simulink model "sampleModel1407_1_sub_sub"  (R2023a)
settings: Solver=VariableStepAuto  StartTime=0.0  StopTime=10.0  RelTol=1e-3
libraries: hdlsllib x1
settings Model: Creator=user1  LastModifiedBy=user1
settings OptimizationCC: BlockReduction=off  ConditionallyExecuteInputs=off

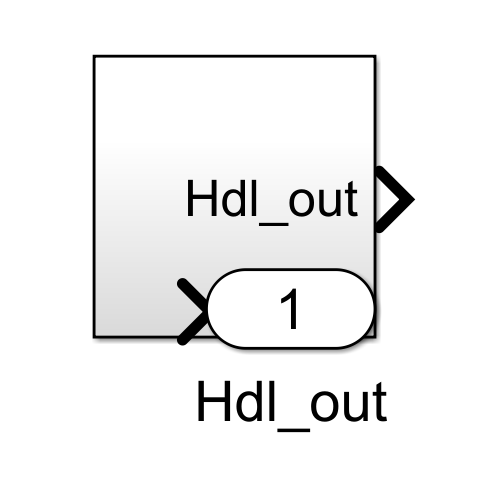
[thumbnail: Simulink's stored preview of the top-level diagram]
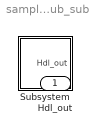
== system sampleModel1407_1_sub_sub ==
  Subsystem : Subsystem
  Hdl_out : Outport  OutDataTypeStr=uint8

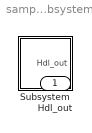
== system sampleModel1407_1_sub_sub/Subsystem ==
  Subsystem : Subsystem
  Hdl_out : Outport  OutDataTypeStr=uint8

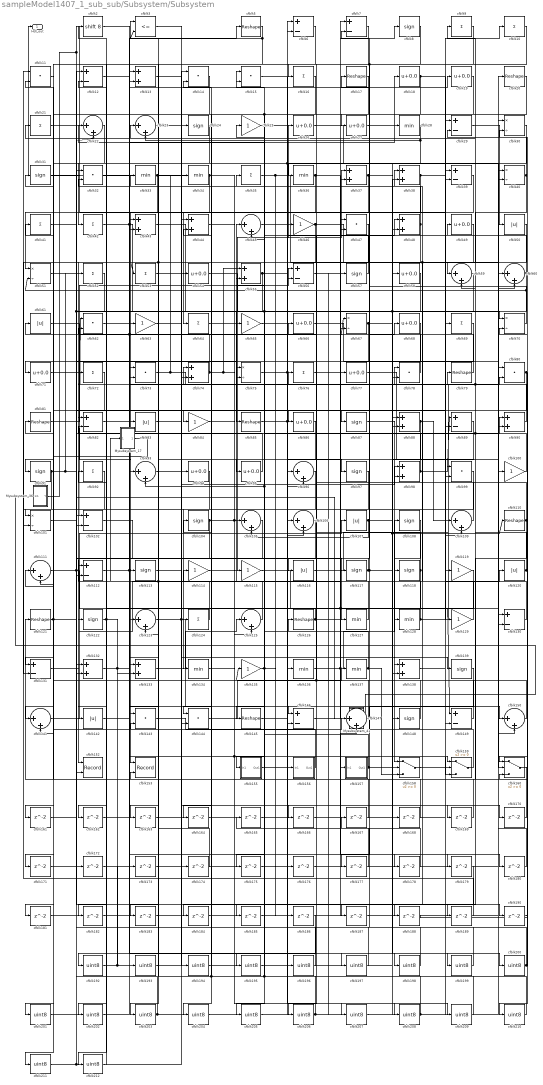
== system sampleModel1407_1_sub_sub/Subsystem/Subsystem ==
  Mysubsystem_17 : Subsystem  TreatAsAtomicUnit=on  RTWFcnName=Mysubsystem_17
      settings: RTWFcnNameOpts=User specified  RTWFileNameOpts=Use function name
  Mysubsystem_36 : Subsystem  TreatAsAtomicUnit=on  RTWFcnName=Mysubsystem_36
      settings: RTWFcnNameOpts=User specified  RTWFileNameOpts=Use function name
  Mysubsystem_41 : Subsystem  TreatAsAtomicUnit=on  RTWFcnName=Mysubsystem_41
      settings: RTWFcnNameOpts=User specified  RTWFileNameOpts=Use function name
  cfblk{9..10,16,21,35,41..42,52..53,64,69,72,76,92,124} (15 alike) : Sum  Inputs=+  OutDataTypeStr=uint8
  cfblk{25,46,63,65,84,100,114..115,119,129,135} (11 alike) : Gain  OutDataTypeStr=uint8
  cfblk{30,40,51,67,70,75,101} (7 alike) : Product  Inputs=*/  OutDataTypeStr=uint8  RndMeth=Zero  SaturateOnIntegerOverflow=on
  cfblk{6..7,12,29,39,56,82,89,102,112,130..131,146,149} (14 alike) : Sum  Inputs=+-  OutDataTypeStr=uint8
  cfblk{8,24,31,57,87,91,97,104,108,113,117..118,122,139,148} (15 alike) : Signum
  cfblk{22..23,45,59..60,93,96,105..106,109,111,123,125,141,147,150} (16 alike) : Sum  Inputs=|++  OutDataTypeStr=uint8
  cfblk{50,61,83,107,116,120,142} (7 alike) : Abs  OutDataTypeStr=uint8  SaturateOnIntegerOverflow=off
  cfblk{11,14..15,32,47,62,73,78,80,99,143..144} (12 alike) : DotProduct  OutDataTypeStr=uint8
  cfblk{5,17,20,79,81,85,110,121,126,145} (10 alike) : Reshape
  cfblk{28,33..34,36,127..128,134,136..137} (9 alike) : MinMax  OutDataTypeStr=uint8
  cfblk{13,37..38,43..44,48,55,74,88,90,98,132..133,138} (14 alike) : Sum  OutDataTypeStr=uint8
  cfblk152 : Record  FileSettingsInternal="{\"entries\":[{\"content\":{\"excelSettings\":{\"content\":{},\"type\":\"Streamout.ExcelSettings\"}},\"type\":\"Streamout.FileSettingStorage\",\"uuid\":\"\"}],\"packageUris\":[\"http:\\/\\/schema.mathworks.com\\/mf0\\/streamout_blocks\\/R2020a\"],\"version\":\"1.0\"}"  Layout=[1 1]  SignalsInternal="{\"entries\":[{\"content\":{\"signals\":[{\"content\":{\"blockPath\":[],\"dimensions\":[1],\"domain\":\"\",\"lineColor\":\"#a2142f\",\"plots\":[1],\"port\":1,\"signalID\":12907,\"signalName\":\"cfblk99\"},\"type\":\"RecordBlkView.Signal\",\"uuid\":\"\"},{\"content\":{\"blockPath\":[],\"dimensions\":[1],\"domain\":\"\",\"lineColor\":\"#139fff\",\"plots\":[1],\"port\":2,\"signalID\":12910,\"signalName\":\"cfblk20\"},\"type\":\"RecordBlkView.Signal\",\"uuid\":\"\"}]},\"type\":\"RecordBlkView.InputSignals\",\"uuid\":\"\"}],\"packageUris\":[\"http:\\/\\/schema.mathworks.com\\/mf0\\/streamout_blocks\\/R2020a\"],\"version\":\"1.0\"}"  VisualizationBindings="{\"xyplotplugin\":{\"info\":[{\"series\":[{\"bindingParametersList\":[{\"parameter\":\"X-Axis\",\"signalID\":12907,\"signalName\":\"cfblk99\"},{\"parameter\":\"Y-Axis\",\"signalID\":12910,\"signalName\":\"cfblk20\"}],\"seriesID\":1819}],\"subplotID\":1}]}}"  CompatibilityTag=XY  st=-1
  cfblk153 : Record  FileSettingsInternal="{\"entries\":[{\"content\":{\"excelSettings\":{\"content\":{},\"type\":\"Streamout.ExcelSettings\"}},\"type\":\"Streamout.FileSettingStorage\",\"uuid\":\"\"}],\"packageUris\":[\"http:\\/\\/schema.mathworks.com\\/mf0\\/streamout_blocks\\/R2020a\"],\"version\":\"1.0\"}"  Layout=[1 1]  SignalsInternal="{\"entries\":[{\"content\":{\"signals\":[{\"content\":{\"blockPath\":[],\"dimensions\":[1],\"domain\":\"\",\"lineColor\":\"#a2142f\",\"plots\":[1],\"port\":1,\"signalID\":12899,\"signalName\":\"cfblk47\"},\"type\":\"RecordBlkView.Signal\",\"uuid\":\"\"},{\"content\":{\"blockPath\":[],\"dimensions\":[1],\"domain\":\"\",\"lineColor\":\"#139fff\",\"plots\":[1],\"port\":2,\"signalID\":12902,\"signalName\":\"cfblk208\"},\"type\":\"RecordBlkView.Signal\",\"uuid\":\"\"}]},\"type\":\"RecordBlkView.InputSignals\",\"uuid\":\"\"}],\"packageUris\":[\"http:\\/\\/schema.mathworks.com\\/mf0\\/streamout_blocks\\/R2020a\"],\"version\":\"1.0\"}"  VisualizationBindings="{\"xyplotplugin\":{\"info\":[{\"series\":[{\"bindingParametersList\":[{\"parameter\":\"X-Axis\",\"signalID\":12899,\"signalName\":\"cfblk47\"},{\"parameter\":\"Y-Axis\",\"signalID\":12902,\"signalName\":\"cfblk208\"}],\"seriesID\":54978}],\"subplotID\":1}]}}"  CompatibilityTag=XY  st=-1
  cfblk155 : Subsystem
      settings: LibrarySourceBlock=|
      | hdlsllib/Ports &
      | Subsystems/Subsystem
  cfblk156 : Subsystem
      settings: LibrarySourceBlock=|
      | hdlsllib/Ports &
      | Subsystems/Subsystem
  cfblk157 : Subsystem
      settings: LibrarySourceBlock=|
      | hdlsllib/Ports &
      | Subsystems/Subsystem
  cfblk158 : Switch  OutDataTypeStr=uint8  SaturateOnIntegerOverflow=off  InputSameDT=off
  cfblk159 : Switch  OutDataTypeStr=uint8  SaturateOnIntegerOverflow=off  InputSameDT=off
  cfblk160 : Switch  OutDataTypeStr=uint8  SaturateOnIntegerOverflow=off  InputSameDT=off
  cfblk{161..190} (30 alike) : Delay  SampleTime=1
  cfblk{18..19,26..27,49,54,58,66,68,71,77,86,94..95} (14 alike) : Bias  Bias=0.0  SaturateOnIntegerOverflow=off
  cfblk{192..212} (21 alike) : DataTypeConversion  OutDataTypeStr=uint8  SaturateOnIntegerOverflow=off  RndMeth=Floor
  cfblk2 : ArithShift  BitShiftNumber=8
  cfblk3 : RelationalOperator  Operator=<=  OutDataTypeStr=boolean  InputSameDT=off
  Hdl_out : Outport  OutDataTypeStr=uint8
  wires:
  Mysubsystem_41/1(Out1) -> Mysubsystem_36/1(In1)
  Mysubsystem_36/1(Y) -> cfblk64/1, cfblk75/1
  Mysubsystem_17/1(Out1) -> cfblk161/1
  cfblk125/1 -> Mysubsystem_17/1(In1)
  cfblk212/1 -> cfblk92/1
  cfblk16/1 -> cfblk212/1
  cfblk211/1 -> cfblk22/2, cfblk94/1
  cfblk210/1 -> cfblk44/2
  cfblk209/1 -> cfblk44/1
  cfblk165/1 -> cfblk209/1
  cfblk208/1 -> cfblk14/2, cfblk153/2, cfblk75/2, cfblk20/1
  cfblk207/1 -> cfblk69/1
  cfblk206/1 -> cfblk123/2, cfblk57/1
  cfblk205/1 -> cfblk96/2
  cfblk204/1 -> cfblk96/1
  cfblk179/1 -> cfblk204/1
  cfblk203/1 -> cfblk132/1, cfblk148/1
  cfblk202/1 -> cfblk13/2
  cfblk186/1 -> cfblk202/1
  cfblk201/1 -> cfblk13/1
  cfblk11/1 -> cfblk201/1
  cfblk200/1 -> cfblk165/1, cfblk30/2
  cfblk199/1 -> cfblk65/1
  cfblk198/1 -> cfblk167/1
  cfblk65/1 -> cfblk198/1
  cfblk197/1 -> cfblk12/2
  cfblk196/1 -> cfblk12/1
  cfblk145/1 -> cfblk196/1
  cfblk195/1 -> cfblk168/1
  cfblk12/1 -> cfblk195/1
  cfblk194/1 -> cfblk106/2
  cfblk3/1 -> cfblk194/1
  cfblk193/1 -> cfblk106/1
  cfblk192/1 -> cfblk174/1, cfblk173/1
  cfblk190/1 -> cfblk160/3
  cfblk189/1 -> cfblk11/1
  cfblk188/1 -> cfblk160/1
  cfblk187/1 -> cfblk39/1
  cfblk185/1 -> cfblk88/1
  cfblk184/1 -> cfblk60/1
  cfblk183/1 -> cfblk144/2
  cfblk182/1 -> cfblk147/2
  cfblk119/1 -> cfblk182/1
  cfblk181/1 -> cfblk80/1
  cfblk180/1 -> cfblk40/1
  cfblk63/1 -> cfblk180/1
  cfblk178/1 -> cfblk15/2
  cfblk76/1 -> cfblk178/1
  cfblk177/1 -> cfblk45/2
  cfblk139/1 -> cfblk177/1
  cfblk176/1 -> cfblk109/2
  cfblk175/1 -> cfblk158/2
  cfblk174/1 -> cfblk143/2
  cfblk173/1 -> cfblk30/1
  cfblk172/1 -> cfblk62/2
  cfblk51/1 -> cfblk172/1
  cfblk171/1 -> cfblk74/2
  cfblk24/1 -> cfblk171/1
  cfblk170/1 -> cfblk59/2
  cfblk169/1 -> cfblk111/1
  cfblk168/1 -> cfblk14/1
  cfblk167/1 -> cfblk102/1
  cfblk166/1 -> cfblk149/2
  cfblk83/1 -> cfblk166/1
  cfblk164/1 -> cfblk56/2
  cfblk163/1 -> cfblk48/2
  cfblk105/1 -> cfblk163/1
  cfblk162/1 -> cfblk73/1
  cfblk161/1 -> cfblk32/1
  cfblk93/1 -> cfblk138/1
  cfblk121/1 -> cfblk81/1, cfblk90/2
  cfblk107/1 -> cfblk105/2, cfblk170/1
  cfblk66/1 -> cfblk150/2
  cfblk17/1 -> cfblk36/1
  cfblk39/1 -> cfblk142/1
  cfblk23/1 -> cfblk24/1
  cfblk86/1 -> cfblk133/1
  cfblk33/1 -> cfblk43/2, cfblk88/2
  cfblk137/1 -> cfblk25/1, cfblk93/2, cfblk158/3
  cfblk71/1 -> cfblk38/2
  cfblk27/1 -> cfblk18/1
  cfblk89/1 -> cfblk95/1
  cfblk48/1 -> cfblk32/2, cfblk124/1
  cfblk148/1 -> cfblk135/1, cfblk126/1
  cfblk25/1 -> cfblk97/1
  cfblk135/1 -> cfblk175/1, cfblk176/1
  cfblk40/1 -> cfblk59/1, cfblk29/2
  cfblk91/1 -> Mysubsystem_41/1(In1), cfblk52/1, cfblk131/2
  cfblk43/1 -> cfblk105/1
  cfblk64/1 -> cfblk26/1
  cfblk53/1 -> cfblk99/2
  cfblk19/1 -> cfblk54/1, cfblk205/1
  cfblk100/1 -> cfblk49/1, cfblk46/1
  cfblk144/1 -> cfblk137/1
  cfblk13/1 -> cfblk200/1
  cfblk156/1(Out1) -> cfblk41/1
  cfblk67/1 -> cfblk99/1, cfblk145/1
  cfblk106/1 -> cfblk192/1
  cfblk57/1 -> cfblk22/1
  cfblk5/1 -> cfblk73/2, cfblk3/2
  cfblk9/1 -> cfblk87/1, cfblk112/1
  cfblk58/1 -> cfblk117/1
  cfblk84/1 -> cfblk115/1
  cfblk80/1 -> cfblk162/1, cfblk210/1
  cfblk77/1 -> cfblk130/1
  cfblk114/1 -> cfblk29/1
  cfblk20/1 -> cfblk152/2
  cfblk129/1 -> cfblk104/1
  cfblk90/1 -> cfblk78/1
  cfblk113/1 -> cfblk98/2
  cfblk56/1 -> cfblk48/1
  cfblk98/1 -> cfblk89/1, cfblk35/1
  cfblk61/1 -> cfblk93/1
  cfblk2/1 -> cfblk43/1
  cfblk68/1 -> cfblk131/1
  cfblk14/1 -> cfblk91/1
  cfblk131/1 -> cfblk7/1
  cfblk30/1 -> cfblk111/2
  cfblk101/1 -> cfblk116/1
  cfblk155/1(Out1) -> cfblk98/1
  cfblk138/1 -> cfblk120/1
  cfblk97/1 -> cfblk141/2
  cfblk95/1 -> cfblk2/1
  cfblk46/1 -> cfblk101/1, cfblk60/2
  cfblk108/1 -> cfblk118/1
  cfblk52/1 -> cfblk102/2
  cfblk130/1 -> cfblk38/1
  cfblk132/1 -> cfblk133/2, cfblk179/1
  cfblk42/1 -> cfblk85/1, cfblk28/1
  cfblk15/1 -> cfblk40/2, cfblk169/1
  cfblk159/1 -> cfblk114/1
  cfblk158/1 -> cfblk39/2
  cfblk116/1 -> cfblk90/1
  cfblk142/1 -> cfblk79/1
  cfblk54/1 -> cfblk70/1
  cfblk31/1 -> cfblk129/1
  cfblk82/1 -> cfblk67/1, cfblk19/1
  cfblk126/1 -> cfblk139/1, cfblk123/1
  cfblk150/1 -> cfblk76/1
  cfblk115/1 -> cfblk128/1
  cfblk55/1 -> cfblk156/1(In1), cfblk132/2
  cfblk96/1 -> cfblk203/1
  cfblk59/1 -> cfblk144/1
  cfblk75/1 -> cfblk6/2, cfblk159/1
  cfblk92/1 -> cfblk211/1
  cfblk88/1 -> cfblk109/1, cfblk164/1
  cfblk109/1 -> cfblk74/1
  cfblk22/1 -> cfblk71/1
  cfblk136/1 -> cfblk108/1, cfblk8/1
  cfblk74/1 -> cfblk55/1, cfblk207/1, cfblk11/2
  cfblk38/1 -> cfblk10/1, cfblk184/1
  cfblk45/1 -> cfblk6/1
  cfblk18/1 -> cfblk119/1, cfblk183/1
  cfblk32/1 -> cfblk146/1
  cfblk111/1 -> cfblk149/1, cfblk157/1(In1), cfblk190/1
  cfblk112/1 -> cfblk15/1, cfblk159/2
  cfblk149/1 -> cfblk31/1
  cfblk146/1 -> cfblk68/1
  cfblk28/1 -> cfblk23/2, cfblk78/2
  cfblk124/1 -> cfblk62/1, cfblk3/1
  cfblk26/1 -> cfblk160/2
  cfblk102/1 -> cfblk127/1
  cfblk78/1 -> cfblk17/1
  cfblk117/1 -> cfblk130/2, cfblk47/2, cfblk113/1
  cfblk157/1(Out1) -> cfblk58/1, cfblk110/1, cfblk55/2
  cfblk70/1 -> cfblk37/2, cfblk51/2
  cfblk41/1 -> cfblk84/1, cfblk67/2
  cfblk87/1 -> cfblk158/1
  cfblk50/1 -> cfblk101/2, cfblk188/1
  cfblk104/1 -> cfblk37/1, cfblk197/1, cfblk112/2
  cfblk110/1 -> cfblk66/1, cfblk189/1
  cfblk62/1 -> cfblk5/1
  cfblk49/1 -> cfblk122/1
  cfblk141/1 -> cfblk107/1
  cfblk120/1 -> cfblk23/1, cfblk72/1, cfblk70/2
  cfblk21/1 -> cfblk77/1
  cfblk134/1 -> cfblk159/3, cfblk187/1
  cfblk99/1 -> cfblk152/1
  cfblk34/1 -> cfblk51/1, cfblk125/2, Hdl_out/1
  cfblk60/1 -> cfblk82/1, cfblk185/1, cfblk138/2, cfblk21/1
  cfblk7/1 -> cfblk86/1
  cfblk37/1 -> cfblk83/1, cfblk53/1, cfblk199/1
  cfblk69/1 -> cfblk206/1
  cfblk29/1 -> cfblk50/1
  cfblk147/1 -> cfblk33/1
  cfblk85/1 -> cfblk136/1, cfblk47/1
  cfblk72/1 -> cfblk141/1
  cfblk35/1 -> cfblk100/1, cfblk186/1
  cfblk6/1 -> cfblk143/1
  cfblk73/1 -> cfblk80/2, cfblk34/1
  cfblk122/1 -> cfblk82/2, cfblk193/1
  cfblk44/1 -> cfblk208/1
  cfblk10/1 -> cfblk27/1, cfblk181/1
  cfblk94/1 -> cfblk134/1
  cfblk133/1 -> cfblk125/1
  cfblk81/1 -> cfblk56/1
  cfblk143/1 -> cfblk147/1
  cfblk160/1 -> cfblk121/1
  cfblk118/1 -> cfblk61/1, cfblk155/1(In1)
  cfblk8/1 -> cfblk16/1
  cfblk127/1 -> cfblk45/1
  cfblk128/1 -> cfblk9/1, cfblk7/2
  cfblk79/1 -> cfblk42/1
  cfblk36/1 -> cfblk63/1, cfblk89/2
  cfblk47/1 -> cfblk153/1
  cfblk123/1 -> cfblk150/1, cfblk146/2

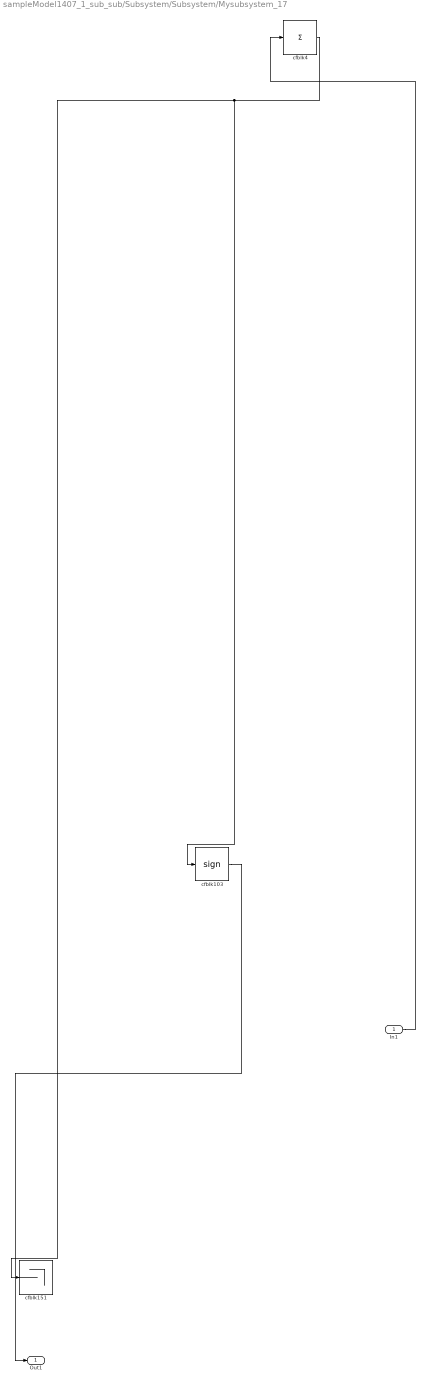
== system sampleModel1407_1_sub_sub/Subsystem/Subsystem/Mysubsystem_17 ==
  In1 : Inport
  cfblk103 : Signum
  cfblk151 : Terminator
  cfblk4 : Sum  Inputs=+
  Out1 : Outport
  wires:
  cfblk4/1 -> cfblk103/1, cfblk151/1
  cfblk103/1 -> Out1/1
  In1/1 -> cfblk4/1

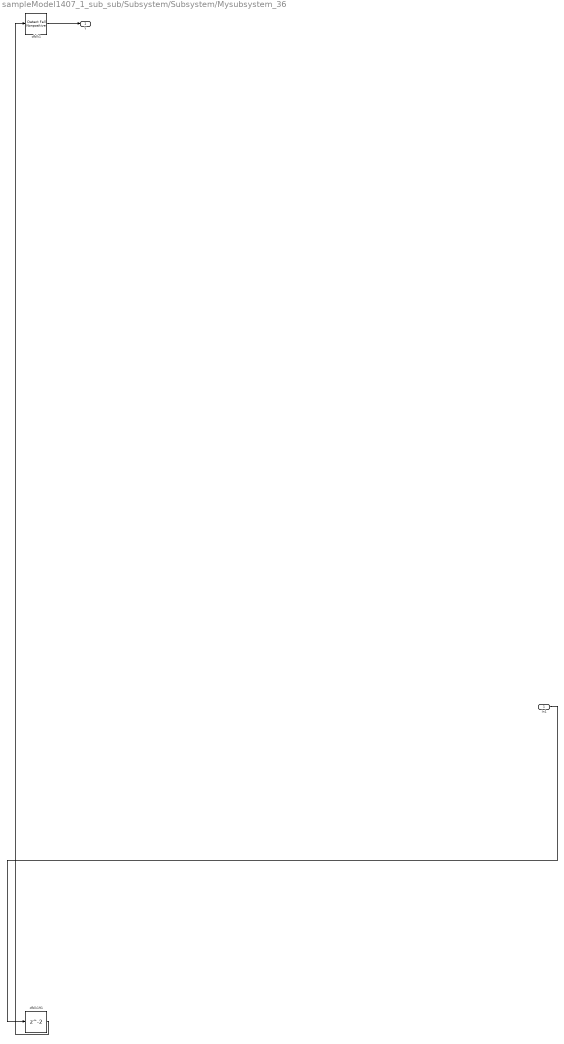
== system sampleModel1407_1_sub_sub/Subsystem/Subsystem/Mysubsystem_36 ==
  In1 : Inport
  cfblk1 : hdlsllib/Logic and Bit Operations/Detect Fall Nonpositive  vinit=0  OutDataTypeStr=boolean
  cfblk191 : Delay  SampleTime=1
  Y : Outport
  wires:
  cfblk191/1 -> cfblk1/1
  cfblk1/1 -> Y/1
  In1/1 -> cfblk191/1

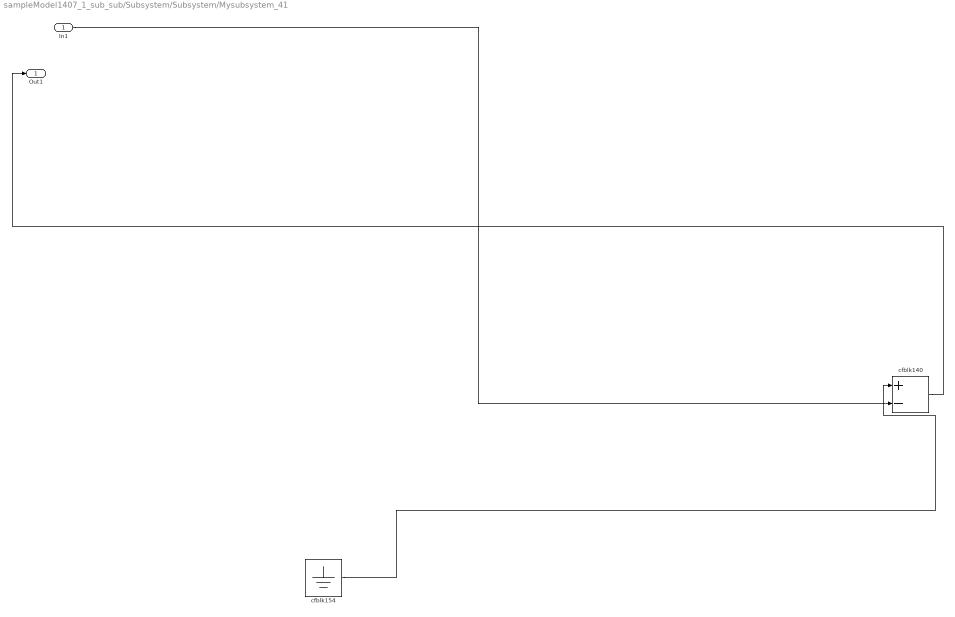
== system sampleModel1407_1_sub_sub/Subsystem/Subsystem/Mysubsystem_41 ==
  In1 : Inport
  cfblk140 : Sum  Inputs=+-
  cfblk154 : Ground
  Out1 : Outport
  wires:
  cfblk154/1 -> cfblk140/1
  cfblk140/1 -> Out1/1
  In1/1 -> cfblk140/2

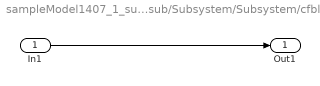
== system sampleModel1407_1_sub_sub/Subsystem/Subsystem/cfblk155 ==
  In1 : Inport
  Out1 : Outport
  wires:
  In1/1 -> Out1/1

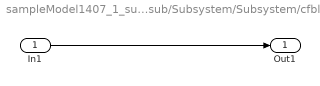
== system sampleModel1407_1_sub_sub/Subsystem/Subsystem/cfblk156 ==
  In1 : Inport
  Out1 : Outport
  wires:
  In1/1 -> Out1/1

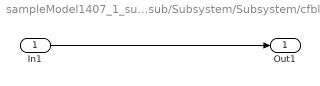
== system sampleModel1407_1_sub_sub/Subsystem/Subsystem/cfblk157 ==
  In1 : Inport
  Out1 : Outport
  wires:
  In1/1 -> Out1/1
